simulink model "c"  (R2023a)
settings: Solver=ode4  StartTime=0.0  StopTime=15  FixedStep=0.002  RelTol=1e-3
InitFcn:
  | init;
values from neighbouring files (symbols this model uses):
  g = 9.81    [init.m]
  N = 4    [init.m]
  T = [0.25, 0.5, 1]    [c_T_vary.m]    (also in init.m = 0.5)
  t_f = 15    [init.m]
  v_c = 1300    [init.m]
settings Model: Creator=Ali  LastModifiedBy=Ali

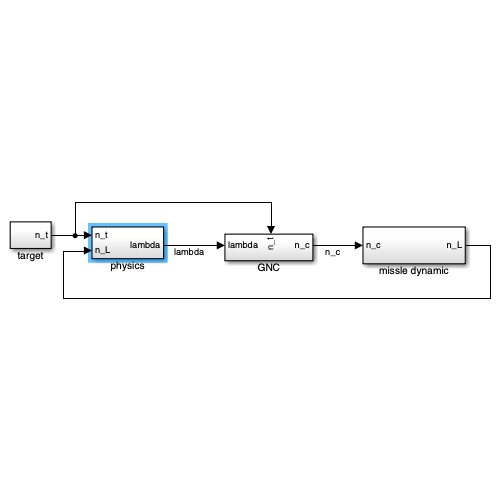
[thumbnail: Simulink's stored preview of the top-level diagram]
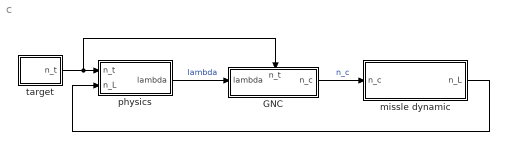
== system c ==
  GNC : Subsystem
      settings: PortSchema="{\"entries\":[{\"content\":{\"sides\":[{\"content\":{\"connectorIds\":[\"In1\"]},\"type\":\"ConnectorPlacement.EquallySpacedRectSide\",\"uuid\":\"ed75f11e-c865-4004-9925-7377fa04d387\"},{\"content\":{\"connectorIds\":[\"Out1\"],\"side\":\"RIGHT\"},\"type\":\"ConnectorPlacement.EquallySpacedRectSide\",\"uuid\":\"bae2f0f6-1e21-4a13-88c5-2ae7c6156ea9\"},{\"content\":{\"connectorIds\":[\"In2\"],\"side\":\"TOP\"},\"type\":\"ConnectorPlacement.EquallySpacedRectSide\",\"uuid\":\"941d1b82-2a2d-4b33-9910-844af34ed272\"}]},\"type\":\"ConnectorPlacement.EquallySpacedConnector\",\"uuid\":\"c15f6690-1bd4-4323-98c9-9e5b3f44ccd0\"}],\"packageUris\":[\"http://schema.mathworks.com/mf0/Connector/R2020b\"],\"version\":\"1.0\"}"
  missle dynamic : Subsystem
  physics : Subsystem
  target : Subsystem
  wires:
  target/1(n_t) -> GNC/2(n_t), physics/1(n_t)
  physics/1(lambda) -> GNC/1(lambda)  "lambda"
  GNC/1(n_c) -> missle dynamic/1(n_c)  "n_c"
  missle dynamic/1(n_L) -> physics/2(n_L)

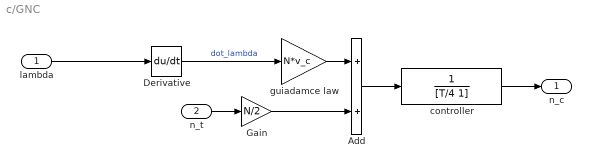
== system c/GNC ==
  lambda : Inport
  n_t : Inport  Port=2
  Add : Sum
  Derivative : Derivative
  Gain : Gain  Gain=N/2
  controller : TransferFcn  Denominator=[T/4 1]
  guiadamce law : Gain  Gain=N*v_c
  n_c : Outport
  wires:
  lambda/1 -> Derivative/1
  Derivative/1 -> guiadamce law/1  "dot_lambda"
  n_t/1 -> Gain/1
  guiadamce law/1 -> Add/1
  Gain/1 -> Add/2
  Add/1 -> controller/1
  controller/1 -> n_c/1

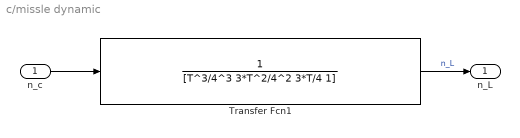
== system c/missle dynamic ==
  n_c : Inport
  Transfer Fcn1 : TransferFcn  Denominator=[T^3/4^3 3*T^2/4^2 3*T/4 1]
  n_L : Outport
  wires:
  Transfer Fcn1/1 -> n_L/1  "n_L"
  n_c/1 -> Transfer Fcn1/1

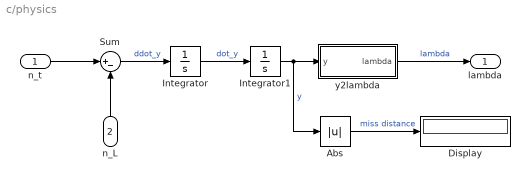
== system c/physics ==
  n_t : Inport
  n_L : Inport  Port=2
  Abs : Abs  SaturateOnIntegerOverflow=off
  Display : Display
  Integrator : Integrator
  Integrator1 : Integrator
  Sum : Sum  Inputs=|+-
  y2lambda : Subsystem
  lambda : Outport
  wires:
  Sum/1 -> Integrator/1  "ddot_y"
  n_t/1 -> Sum/1
  n_L/1 -> Sum/2
  y2lambda/1(lambda) -> lambda/1  "lambda"
  Integrator/1 -> Integrator1/1  "dot_y"
  Integrator1/1 -> Abs/1, y2lambda/1(y)  "y"
  Abs/1 -> Display/1  "miss distance"

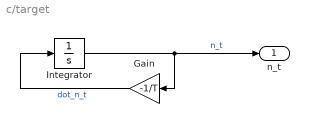
== system c/target ==
  Gain : Gain  Gain=-1/T
  Integrator : Integrator  InitialCondition=3*g
  n_t : Outport
  wires:
  Gain/1 -> Integrator/1  "dot_n_t"
  Integrator/1 -> n_t/1, Gain/1  "n_t"

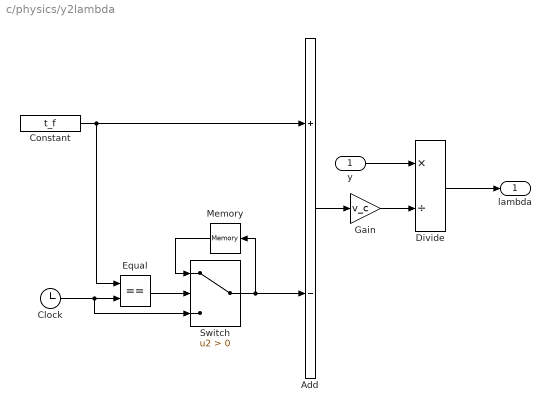
== system c/physics/y2lambda ==
  y : Inport
  Add : Sum  Inputs=+-
  Clock : Clock
  Constant : Constant  Value=t_f
  Divide : Product  Inputs=*/
  Equal : RelationalOperator  Operator===  OutDataTypeStr=boolean  RndMeth=Simplest  InputSameDT=off
  Gain : Gain  Gain=v_c
  Memory : Memory
  Switch : Switch  Criteria=u2 > Threshold  SaturateOnIntegerOverflow=off  InputSameDT=off
  lambda : Outport
  wires:
  Divide/1 -> lambda/1
  y/1 -> Divide/1
  Gain/1 -> Divide/2
  Constant/1 -> Add/1, Equal/1
  Clock/1 -> Switch/3, Equal/2
  Equal/1 -> Switch/2
  Memory/1 -> Switch/1
  Switch/1 -> Add/2, Memory/1
  Add/1 -> Gain/1
